simulink model "bdotSim"  (R2025a)
settings: Solver=FixedStepAuto  StartTime=0.0  StopTime=12000  FixedStep=5  RelTol=1e-3
undefined symbols (not defined in the file or in its folder): IAU
libraries: matrix_library x1, aerolibtransform2 x1
settings Model: Creator=cdwy3  LastModifiedBy=cdwy3

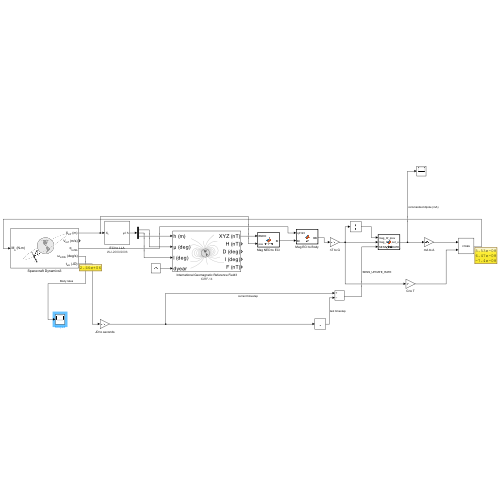
[thumbnail: Simulink's stored preview of the top-level diagram]
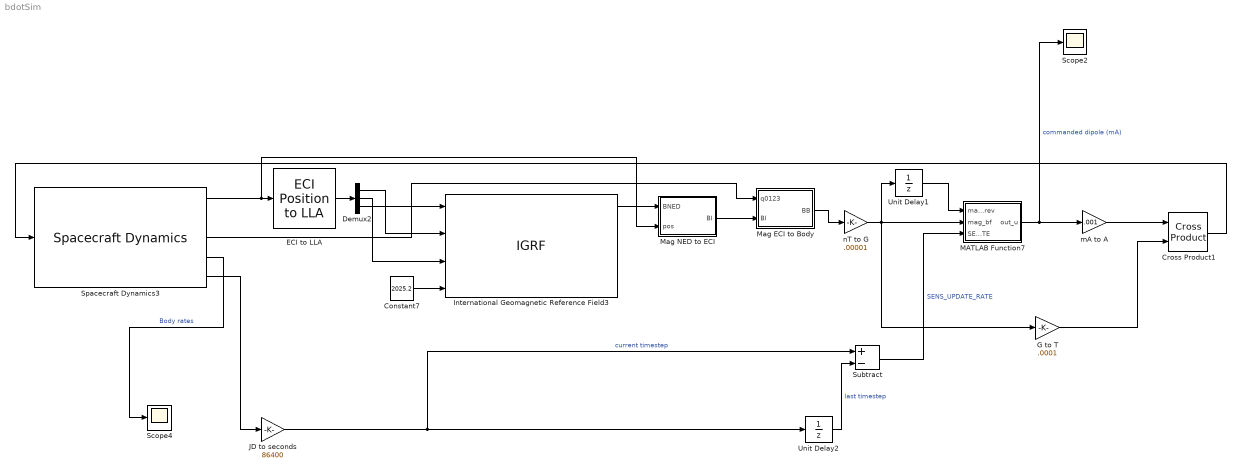
== system bdotSim ==
  Constant7 : Constant  Value=2025.2
  Cross Product1 : matrix_library/Cross Product
  Demux2 : Demux  Outputs=3
  ECI to LLA : aerolibtransform2/ECI Position to LLA  red=IAU-2000/2006  year=2013  month=January  day=1  hour=0  min=0  sec=0  deltaT=None  errorflag=Error  extraparamflag=off  eunits=Metric (MKS)  earthmodel=WGS84  flat=1/298.257223563  eqradius=6378137
      settings: AttributesFormatString=%<red>
  G to T : Gain  Gain=.0001
  International Geomagnetic Reference Field3 : IGRF  month=January  day=1  sv_out=off
      settings: AttributesFormatString=%<generation>
  JD to seconds : Gain  Gain=86400
  MATLAB Function7 : MATLAB Function  TreatAsAtomicUnit=on
  Mag ECI to Body : MATLAB Function  TreatAsAtomicUnit=on
  Mag NED to ECI : MATLAB Function  TreatAsAtomicUnit=on
  Scope2 : Scope
      settings: DataLoggingVariableName=ScopeData2
  Scope4 : Scope
      settings: ActiveDisplayYMinimum=-4.7437885423070316  ActiveDisplayYMaximum=5.1934915160474038  YLabel=Body Rates (deg/s)  DataLoggingVariableName=ScopeData4
  Spacecraft Dynamics3 : SpacecraftDynamics  forcesIn=off  startDate=2460438.0  mass=9.0  inertia=[0.0797 -0.00005 0.00125 ;-0.00005 0.1291 -0.00103;0.00125 -0.00103 0.1310]  orbitType=Circular inclined  semiMajorAxis=6821000  eccentricity=0  inclination=55  raan=0  argPeriapsis=0  trueAnomaly=0  attitudeRate=[3 3 3]  useGravGrad=off
  Subtract : Sum  Inputs=+-
  Unit Delay1 : UnitDelay  SampleTime=-1  HasFrameUpgradeWarning=on
  Unit Delay2 : UnitDelay  SampleTime=-1  HasFrameUpgradeWarning=on
  mA to A : Gain  Gain=.001
  nT to G : Gain  Gain=.00001
  wires:
  Constant7/1 -> International Geomagnetic Reference Field3/4
  Spacecraft Dynamics3/1 -> ECI to LLA/1, Mag NED to ECI/2(pos)
  International Geomagnetic Reference Field3/1 -> Mag NED to ECI/1(BNED)
  Mag NED to ECI/1(BI) -> Mag ECI to Body/2(BI)
  Spacecraft Dynamics3/3 -> Mag ECI to Body/1(q0123)
  Mag ECI to Body/1(BB) -> nT to G/1
  Unit Delay1/1 -> MATLAB Function7/1(mag_bf_prev)
  MATLAB Function7/1(out_u) -> Scope2/1, mA to A/1  "commanded dipole (mA)"
  mA to A/1 -> Cross Product1/1
  G to T/1 -> Cross Product1/2
  nT to G/1 -> Unit Delay1/1, MATLAB Function7/2(mag_bf), G to T/1
  Spacecraft Dynamics3/4 -> Scope4/1  "Body rates"
  Spacecraft Dynamics3/5 -> JD to seconds/1
  Unit Delay2/1 -> Subtract/2  "last timestep"
  Subtract/1 -> MATLAB Function7/3(SENS_UPDATE_RATE)  "SENS_UPDATE_RATE"
  JD to seconds/1 -> Subtract/1, Unit Delay2/1  "current timestep"
  Cross Product1/1 -> Spacecraft Dynamics3/1
  ECI to LLA/1 -> Demux2/1
  Demux2/1 -> International Geomagnetic Reference Field3/2
  Demux2/2 -> International Geomagnetic Reference Field3/3
  Demux2/3 -> International Geomagnetic Reference Field3/1

== matlab function bdotSim/Mag NED to ECI ==
  data: BNED input; BI output; pos input
function BI = NED2I(BNED,pos)

rvec = [pos(1); pos(2); pos(3)];
rho = norm(rvec);

phi=0;
theta = acos(pos(3) / rho);
psi = atan2(pos(2), pos(1));

ct = cos(theta);
st = sin(theta);
sp = sin(phi);
cp = cos(phi);
ss = sin(psi);
cs = cos(psi);

BI = [ct*cs,sp*st*cs-cp*ss,cp*st*cs+sp*ss;
    ct*ss,sp*st*ss+cp*cs,cp*st*ss-sp*cs;
    -st,sp*ct,cp*ct] * BNED;

== matlab function bdotSim/Mag ECI to Body ==
  data: q0123 input; BB output; BI input
function BB = I2B(q0123,BI)
%compute R such that v(inertial) = TIB v(body)

q0 = q0123(1);
q1 = q0123(2);
q2 = q0123(3);
q3 = q0123(4);

BB = [(q0^2+q1^2-q2^2-q3^2) 2*(q1*q2-q0*q3)  2*(q0*q2+q1*q3);
      2*(q1*q2+q0*q3) (q0^2-q1^2+q2^2-q3^2) 2*(q2*q3-q0*q1);
      2*(q1*q3-q0*q2) 2*(q0*q1+q2*q3) (q0^2-q1^2-q2^2+q3^2)]' * BI;
% Matrix originally adopted from Boom 2010 - Mark Costello
% Copyright - Carlos Montalvo 2015
% You may freely distribute this file but please keep my name in here
% as the original owner

== matlab function bdotSim/MATLAB Function7 ==
  data: mag_bf_prev input; out_u output; mag_bf input; SENS_UPDATE_RATE input
function out_u = bdot(mag_bf_prev,mag_bf,SENS_UPDATE_RATE)

detumble_gain = 5000;
mag_bf_rate = (mag_bf - mag_bf_prev)/SENS_UPDATE_RATE;

out_u = -detumble_gain * mag_bf_rate;  % Control law taken from flight code

% Saturate to ±100 mA·m^2 (0.1 A·m^2)
max_dipole = 100;  % milli-A·m^2
for i = 1:3
        if out_u(i) > max_dipole
            out_u(i) = max_dipole;
        elseif out_u(i) < -max_dipole
            out_u(i) = -max_dipole;
        end
end
